simulink model "DOF4_model_v2"  (R2023a)
settings: Solver=FixedStepAuto  StartTime=0.0  StopTime=10.0  FixedStep=5e-3  RelTol=1e-3
values from neighbouring files (symbols this model uses):
  z_r_type = 1    [DOF_4_parameters.m]
undefined symbols (not defined in the file or in its folder): chassis, constants, suspension
libraries: simulink x1
settings Model: Creator=Cassio de Freitas  LastModifiedBy=Cassio de Freitas
settings DataIOCC: ReturnWorkspaceOutputsName=simout

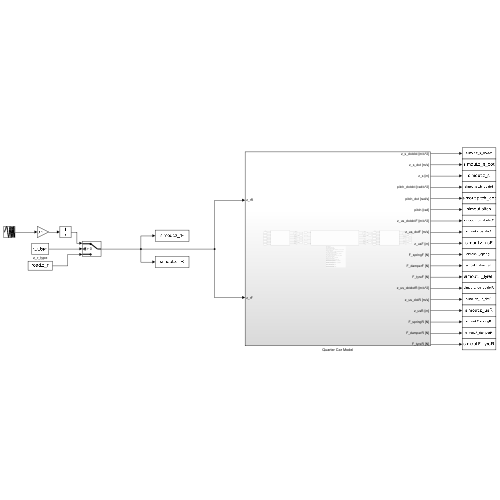
[thumbnail: Simulink's stored preview of the top-level diagram]
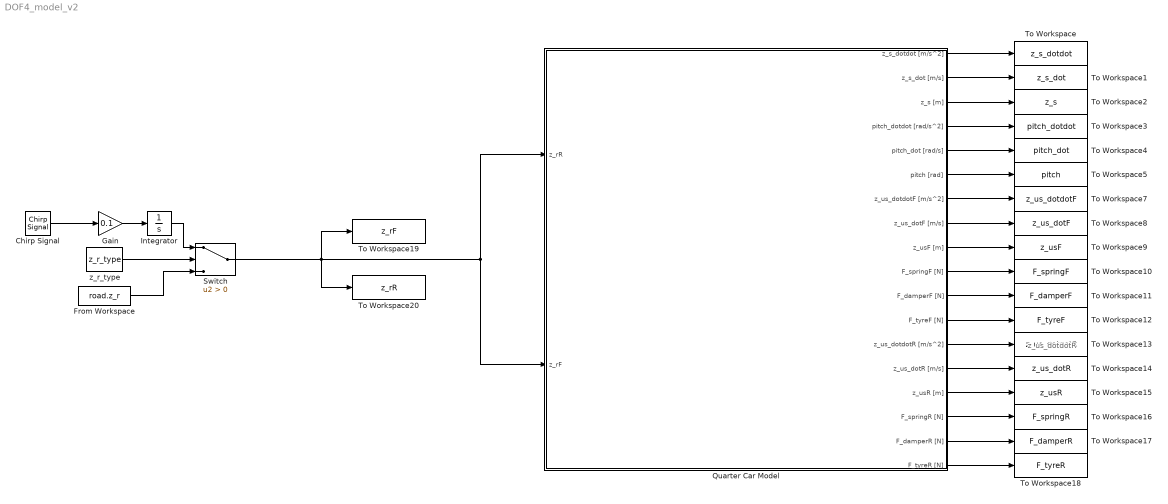
== system DOF4_model_v2 ==
  note: z_us_dotdotR
  Chirp Signal : simulink/Sources/Chirp Signal  f1=0.1  T=100  f2=50
  From Workspace : FromWorkspace  VariableName=road.z_r
  Gain : Gain  Gain=0.1
  Integrator : Integrator
  Quarter Car Model : Subsystem
  Switch : Switch  Criteria=u2 > Threshold  SaturateOnIntegerOverflow=off  InputSameDT=off
  To Workspace : ToWorkspace  VariableName=z_s_dotdot  SaveFormat=Timeseries  SampleTime=-1
  To Workspace1 : ToWorkspace  VariableName=z_s_dot  SaveFormat=Timeseries  SampleTime=-1
  To Workspace10 : ToWorkspace  VariableName=F_springF  SaveFormat=Timeseries  SampleTime=-1
  To Workspace11 : ToWorkspace  VariableName=F_damperF  SaveFormat=Timeseries  SampleTime=-1
  To Workspace12 : ToWorkspace  VariableName=F_tyreF  SaveFormat=Timeseries  SampleTime=-1
  To Workspace13 : ToWorkspace  VariableName=z_us_dotdotR  SaveFormat=Timeseries  SampleTime=-1
  To Workspace14 : ToWorkspace  VariableName=z_us_dotR  SaveFormat=Timeseries  SampleTime=-1
  To Workspace15 : ToWorkspace  VariableName=z_usR  SaveFormat=Timeseries  SampleTime=-1
  To Workspace16 : ToWorkspace  VariableName=F_springR  SaveFormat=Timeseries  SampleTime=-1
  To Workspace17 : ToWorkspace  VariableName=F_damperR  SaveFormat=Timeseries  SampleTime=-1
  To Workspace18 : ToWorkspace  VariableName=F_tyreR  SaveFormat=Timeseries  SampleTime=-1
  To Workspace19 : ToWorkspace  VariableName=z_rF  SaveFormat=Timeseries  SampleTime=-1
  To Workspace2 : ToWorkspace  VariableName=z_s  SaveFormat=Timeseries  SampleTime=-1
  To Workspace20 : ToWorkspace  VariableName=z_rR  SaveFormat=Timeseries  SampleTime=-1
  To Workspace3 : ToWorkspace  VariableName=pitch_dotdot  SaveFormat=Timeseries  SampleTime=-1
  To Workspace4 : ToWorkspace  VariableName=pitch_dot  SaveFormat=Timeseries  SampleTime=-1
  To Workspace5 : ToWorkspace  VariableName=pitch  SaveFormat=Timeseries  SampleTime=-1
  To Workspace7 : ToWorkspace  VariableName=z_us_dotdotF  SaveFormat=Timeseries  SampleTime=-1
  To Workspace8 : ToWorkspace  VariableName=z_us_dotF  SaveFormat=Timeseries  SampleTime=-1
  To Workspace9 : ToWorkspace  VariableName=z_usF  SaveFormat=Timeseries  SampleTime=-1
  z_r_type : Constant  Value=z_r_type
  wires:
  Integrator/1 -> Switch/1
  Gain/1 -> Integrator/1
  From Workspace/1 -> Switch/3
  z_r_type/1 -> Switch/2
  Chirp Signal/1 -> Gain/1
  Quarter Car Model/1(z_s_dotdot [m/s^2]) -> To Workspace/1
  Quarter Car Model/2(z_s_dot [m/s]) -> To Workspace1/1
  Quarter Car Model/3(z_s [m]) -> To Workspace2/1
  Quarter Car Model/4(pitch_dotdot [rad/s^2]) -> To Workspace3/1
  Quarter Car Model/5(pitch_dot [rad/s]) -> To Workspace4/1
  Quarter Car Model/6(pitch [rad]) -> To Workspace5/1
  Quarter Car Model/7(z_us_dotdotF [m/s^2]) -> To Workspace7/1
  Quarter Car Model/8(z_us_dotF [m/s]) -> To Workspace8/1
  Quarter Car Model/9(z_usF [m]) -> To Workspace9/1
  Quarter Car Model/10(F_springF [N]) -> To Workspace10/1
  Quarter Car Model/11(F_damperF [N]) -> To Workspace11/1
  Quarter Car Model/12(F_tyreF [N]) -> To Workspace12/1
  Quarter Car Model/13(z_us_dotdotR [m/s^2]) -> To Workspace13/1
  Quarter Car Model/14(z_us_dotR [m/s]) -> To Workspace14/1
  Quarter Car Model/15(z_usR [m]) -> To Workspace15/1
  Quarter Car Model/16(F_springR [N]) -> To Workspace16/1
  Quarter Car Model/17(F_damperR [N]) -> To Workspace17/1
  Quarter Car Model/18(F_tyreR [N]) -> To Workspace18/1
  Switch/1 -> To Workspace20/1, To Workspace19/1, Quarter Car Model/1(z_rR), Quarter Car Model/2(z_rF)

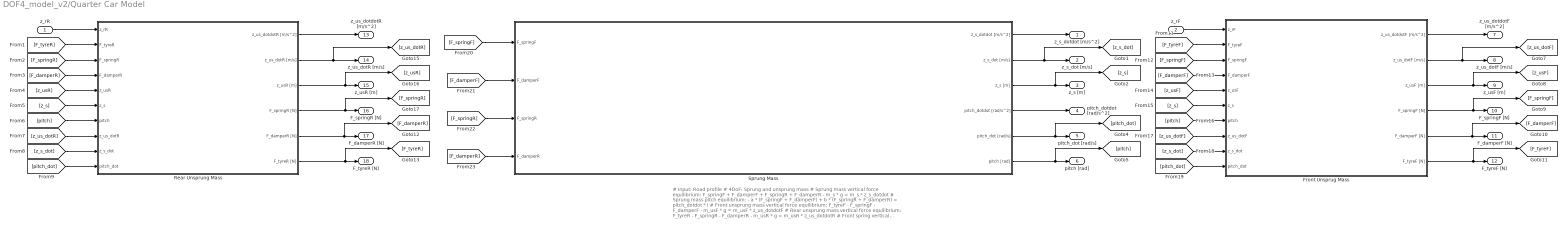
== system DOF4_model_v2/Quarter Car Model ==
  note: # Input: Road profile
      |
      | # 4DoF: Sprung and unsprung mass
      |
      | # Sprung mass vertical force equilibrium:
      | F_springF + F_damperF + F_springR + F_damperR - m_s * g = m_s * z_s_dotdot
      |
      | # Sprung mass pitch equilibrium:
      | - a * (F_springF + F_damperF) + b * (F_springR + F_damperR) = pitch_dotdot * I
      |
      | # Front unsprung mass vertical force equilibrium:
      | F_tyreF - F_springF - F_damperF - m_usF * g = m_usF * z_us_dotdotF
      |
      | # Rear unsprung mass vertical force equilibrium:
      | F_tyreR - F_springR - F_damperR - m_usR * g = m_usR * z_us_dotdotR
      |
      | # Front spring vertical force equilibrium
      | F_springF = (z_usF - (z_s - pitch * a)) * k_springF + F0F
      |
      | # Rear spring vertical force equilibrium
      | F_springR = (z_usR - (z_s + pitch * b)) * k_springR + F0R
      |
      | # Front damper vertical force equilibrium
      | F_damperF = (z_us_dotF - (z_s_dot - pitch_dot * a)) * c_damperF
      |
      | # Rear damper vertical force equilibrium
      | F_damperR = (z_us_dotR - (z_s_dot + pitch_dot * a)) * c_damperR
      |
      | # Front tyre vertical force equilibrium
      | F_tyreF = (z_rF - z_usF +z0_tyreF) * k_tyreF
      |
      | # Rear tyre vertical force equilibrium
      | F_tyreR = (z_rR - z_usR +z0_tyreR) * k_tyreR
  z_rR : Inport
  z_rF : Inport  Port=2
  Front Unsprug Mass : Subsystem
  Rear Unsprung Mass : Subsystem
  Sprung Mass : Subsystem
  z_s_dotdot [m/s^2] : Outport
  z_s_dot [m/s] : Outport  Port=2
  z_s [m] : Outport  Port=3
  pitch_dotdot [rad/s^2] : Outport  Port=4
  pitch_dot [rad/s] : Outport  Port=5
  pitch [rad] : Outport  Port=6
  z_us_dotdotF [m/s^2] : Outport  Port=7
  z_us_dotF [m/s] : Outport  Port=8
  z_usF [m] : Outport  Port=9
  F_springF [N] : Outport  Port=10
  F_damperF [N] : Outport  Port=11
  F_tyreF [N] : Outport  Port=12
  z_us_dotdotR [m/s^2] : Outport  Port=13
  z_us_dotR [m/s] : Outport  Port=14
  z_usR [m] : Outport  Port=15
  F_springR [N] : Outport  Port=16
  F_damperR [N] : Outport  Port=17
  F_tyreR [N] : Outport  Port=18
  wires:
  Sprung Mass/1(z_s_dotdot [m/s^2]) -> z_s_dotdot [m/s^2]/1
  Sprung Mass/2(z_s_dot [m/s]) -> z_s_dot [m/s]/1, [z_s_dot]
  Sprung Mass/3(z_s [m]) -> [z_s], z_s [m]/1
  Sprung Mass/4(pitch_dotdot [rad/s^2]) -> pitch_dotdot [rad/s^2]/1
  Sprung Mass/5(pitch_dot [rad/s]) -> [pitch_dot], pitch_dot [rad/s]/1
  Sprung Mass/6(pitch [rad]) -> [pitch], pitch [rad]/1
  Front Unsprug Mass/6(F_tyreF [N]) -> F_tyreF [N]/1, [F_tyreF]
  Front Unsprug Mass/5(F_damperF [N]) -> F_damperF [N]/1, [F_damperF]
  Front Unsprug Mass/4(F_springF [N]) -> F_springF [N]/1, [F_springF]
  Front Unsprug Mass/3(z_usF [m]) -> z_usF [m]/1, [z_usF]
  Front Unsprug Mass/2(z_us_dotF [m/s]) -> [z_us_dotF], z_us_dotF [m/s]/1
  Front Unsprug Mass/1(z_us_dotdotF [m/s^2]) -> z_us_dotdotF [m/s^2]/1
  Rear Unsprung Mass/3(z_usR [m]) -> z_usR [m]/1, [z_usR]
  Rear Unsprung Mass/4(F_springR [N]) -> F_springR [N]/1, [F_springR]
  Rear Unsprung Mass/5(F_damperR [N]) -> F_damperR [N]/1, [F_damperR]
  Rear Unsprung Mass/2(z_us_dotR [m/s]) -> [z_us_dotR], z_us_dotR [m/s]/1
  Rear Unsprung Mass/6(F_tyreR [N]) -> F_tyreR [N]/1, [F_tyreR]
  Rear Unsprung Mass/1(z_us_dotdotR [m/s^2]) -> z_us_dotdotR [m/s^2]/1
  z_rR/1 -> Rear Unsprung Mass/1(z_rR)
  [pitch_dot] -> Rear Unsprung Mass/10(pitch_dot)
  [z_s_dot] -> Rear Unsprung Mass/9(z_s_dot)
  [z_us_dotR] -> Rear Unsprung Mass/8(z_us_dotR)
  [pitch] -> Rear Unsprung Mass/7(pitch)
  [z_s] -> Rear Unsprung Mass/6(z_s)
  [z_usR] -> Rear Unsprung Mass/5(z_usR)
  [F_damperR] -> Rear Unsprung Mass/4(F_damperR)
  [F_springR] -> Rear Unsprung Mass/3(F_springR)
  [F_tyreR] -> Rear Unsprung Mass/2(F_tyreR)
  [F_damperF] -> Front Unsprug Mass/4(F_damperF)
  [z_us_dotF] -> Front Unsprug Mass/8(z_us_dotF)
  [z_s_dot] -> Front Unsprug Mass/9(z_s_dot)
  z_rF/1 -> Front Unsprug Mass/1(z_rF)
  [F_tyreF] -> Front Unsprug Mass/2(F_tyreF)
  [pitch] -> Front Unsprug Mass/7(pitch)
  [z_s] -> Front Unsprug Mass/6(z_s)
  [F_springF] -> Front Unsprug Mass/3(F_springF)
  [z_usF] -> Front Unsprug Mass/5(z_usF)
  [pitch_dot] -> Front Unsprug Mass/10(pitch_dot)
  [F_springF] -> Sprung Mass/1(F_springF)
  [F_damperF] -> Sprung Mass/2(F_damperF)
  [F_springR] -> Sprung Mass/3(F_springR)
  [F_damperR] -> Sprung Mass/4(F_damperR)

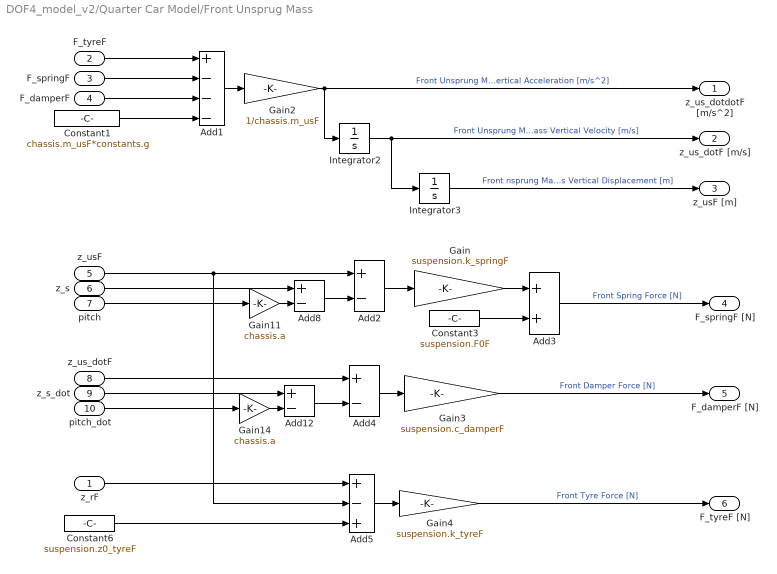
== system DOF4_model_v2/Quarter Car Model/Front Unsprug Mass ==
  z_rF : Inport
  F_tyreF : Inport  Port=2
  F_springF : Inport  Port=3
  F_damperF : Inport  Port=4
  z_usF : Inport  Port=5
  z_s : Inport  Port=6
  pitch : Inport  Port=7
  z_us_dotF : Inport  Port=8
  z_s_dot : Inport  Port=9
  pitch_dot : Inport  Port=10
  Add1 : Sum  Inputs=+---
  Add{2,4,8,12} (4 alike) : Sum  Inputs=+-
  Add3 : Sum
  Add5 : Sum  Inputs=+-+
  Constant1 : Constant  Value=chassis.m_usF*constants.g
  Constant3 : Constant  Value=suspension.F0F
  Constant6 : Constant  Value=suspension.z0_tyreF
  Gain : Gain  Gain=suspension.k_springF
  Gain11 : Gain  Gain=chassis.a
  Gain14 : Gain  Gain=chassis.a
  Gain2 : Gain  Gain=1/chassis.m_usF
  Gain3 : Gain  Gain=suspension.c_damperF
  Gain4 : Gain  Gain=suspension.k_tyreF
  Integrator2 : Integrator
  Integrator3 : Integrator
  z_us_dotdotF [m/s^2] : Outport
  z_us_dotF [m/s] : Outport  Port=2
  z_usF [m] : Outport  Port=3
  F_springF [N] : Outport  Port=4
  F_damperF [N] : Outport  Port=5
  F_tyreF [N] : Outport  Port=6
  wires:
  Integrator3/1 -> z_usF [m]/1  "Front nsprung Mass Vertical Displacement [m]"
  Add1/1 -> Gain2/1
  Integrator2/1 -> z_us_dotF [m/s]/1, Integrator3/1  "Front Unsprung Mass Vertical Velocity [m/s]"
  Gain2/1 -> Integrator2/1, z_us_dotdotF [m/s^2]/1  "Front Unsprung Mass Vertical Acceleration [m/s^2]"
  Gain11/1 -> Add8/2
  z_s/1 -> Add8/1
  Add8/1 -> Add2/2
  Add3/1 -> F_springF [N]/1  "Front Spring Force [N]"
  Gain/1 -> Add3/1
  Add4/1 -> Gain3/1
  Constant3/1 -> Add3/2
  z_usF/1 -> Add5/2, Add2/1
  Gain3/1 -> F_damperF [N]/1  "Front Damper Force [N]"
  Gain14/1 -> Add12/2
  pitch/1 -> Gain11/1
  Add2/1 -> Gain/1
  Add12/1 -> Add4/2
  Add5/1 -> Gain4/1
  z_rF/1 -> Add5/1
  Constant6/1 -> Add5/3
  Gain4/1 -> F_tyreF [N]/1  "Front Tyre Force [N]"
  F_damperF/1 -> Add1/3
  F_tyreF/1 -> Add1/1
  F_springF/1 -> Add1/2
  Constant1/1 -> Add1/4
  z_us_dotF/1 -> Add4/1
  z_s_dot/1 -> Add12/1
  pitch_dot/1 -> Gain14/1

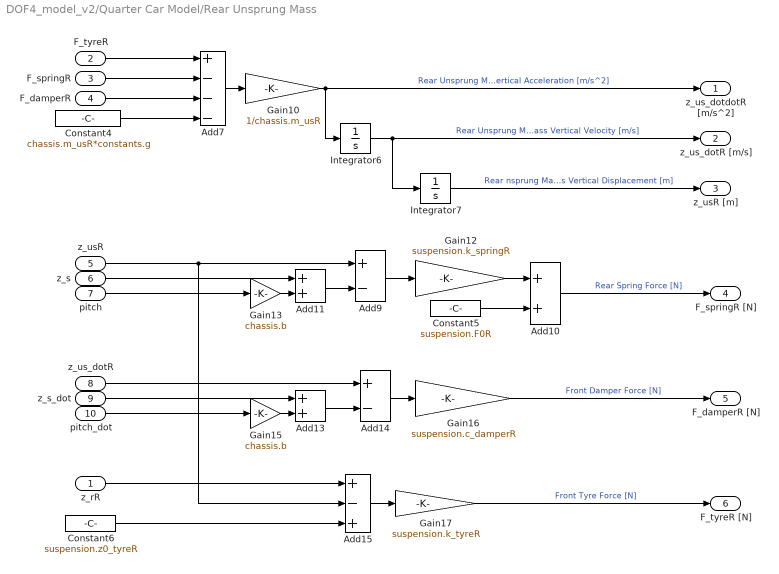
== system DOF4_model_v2/Quarter Car Model/Rear Unsprung Mass ==
  z_rR : Inport
  F_tyreR : Inport  Port=2
  F_springR : Inport  Port=3
  F_damperR : Inport  Port=4
  z_usR : Inport  Port=5
  z_s : Inport  Port=6
  pitch : Inport  Port=7
  z_us_dotR : Inport  Port=8
  z_s_dot : Inport  Port=9
  pitch_dot : Inport  Port=10
  Add10 : Sum
  Add11 : Sum
  Add13 : Sum
  Add14 : Sum  Inputs=+-
  Add15 : Sum  Inputs=+-+
  Add7 : Sum  Inputs=+---
  Add9 : Sum  Inputs=+-
  Constant4 : Constant  Value=chassis.m_usR*constants.g
  Constant5 : Constant  Value=suspension.F0R
  Constant6 : Constant  Value=suspension.z0_tyreR
  Gain10 : Gain  Gain=1/chassis.m_usR
  Gain12 : Gain  Gain=suspension.k_springR
  Gain13 : Gain  Gain=chassis.b
  Gain15 : Gain  Gain=chassis.b
  Gain16 : Gain  Gain=suspension.c_damperR
  Gain17 : Gain  Gain=suspension.k_tyreR
  Integrator6 : Integrator
  Integrator7 : Integrator
  z_us_dotdotR [m/s^2] : Outport
  z_us_dotR [m/s] : Outport  Port=2
  z_usR [m] : Outport  Port=3
  F_springR [N] : Outport  Port=4
  F_damperR [N] : Outport  Port=5
  F_tyreR [N] : Outport  Port=6
  wires:
  Integrator7/1 -> z_usR [m]/1  "Rear nsprung Mass Vertical Displacement [m]"
  Add7/1 -> Gain10/1
  Gain10/1 -> Integrator6/1, z_us_dotdotR [m/s^2]/1  "Rear Unsprung Mass Vertical Acceleration [m/s^2]"
  Integrator6/1 -> z_us_dotR [m/s]/1, Integrator7/1  "Rear Unsprung Mass Vertical Velocity [m/s]"
  Add11/1 -> Add9/2
  Add9/1 -> Gain12/1
  Gain16/1 -> F_damperR [N]/1  "Front Damper Force [N]"
  Add13/1 -> Add14/2
  Gain13/1 -> Add11/2
  Gain12/1 -> Add10/1
  Add14/1 -> Gain16/1
  Add10/1 -> F_springR [N]/1  "Rear Spring Force [N]"
  Gain15/1 -> Add13/2
  Constant5/1 -> Add10/2
  Gain17/1 -> F_tyreR [N]/1  "Front Tyre Force [N]"
  Add15/1 -> Gain17/1
  F_tyreR/1 -> Add7/1
  F_springR/1 -> Add7/2
  F_damperR/1 -> Add7/3
  Constant4/1 -> Add7/4
  z_usR/1 -> Add15/2, Add9/1
  z_s/1 -> Add11/1
  pitch/1 -> Gain13/1
  z_us_dotR/1 -> Add14/1
  z_s_dot/1 -> Add13/1
  pitch_dot/1 -> Gain15/1
  z_rR/1 -> Add15/1
  Constant6/1 -> Add15/3

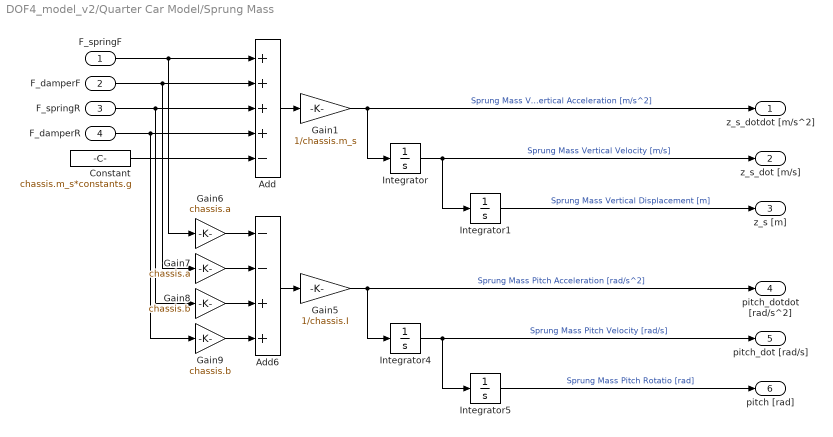
== system DOF4_model_v2/Quarter Car Model/Sprung Mass ==
  F_springF : Inport
  F_damperF : Inport  Port=2
  F_springR : Inport  Port=3
  F_damperR : Inport  Port=4
  Add : Sum  Inputs=++++-
  Add6 : Sum  Inputs=--++
  Constant : Constant  Value=chassis.m_s*constants.g
  Gain1 : Gain  Gain=1/chassis.m_s
  Gain5 : Gain  Gain=1/chassis.I
  Gain6 : Gain  Gain=chassis.a
  Gain7 : Gain  Gain=chassis.a
  Gain8 : Gain  Gain=chassis.b
  Gain9 : Gain  Gain=chassis.b
  Integrator{,1,4..5} (4 alike) : Integrator
  z_s_dotdot [m/s^2] : Outport
  z_s_dot [m/s] : Outport  Port=2
  z_s [m] : Outport  Port=3
  pitch_dotdot [rad/s^2] : Outport  Port=4
  pitch_dot [rad/s] : Outport  Port=5
  pitch [rad] : Outport  Port=6
  wires:
  Integrator4/1 -> pitch_dot [rad/s]/1, Integrator5/1  "Sprung Mass Pitch Velocity [rad/s]"
  Gain5/1 -> pitch_dotdot [rad/s^2]/1, Integrator4/1  "Sprung Mass Pitch Acceleration [rad/s^2]"
  Gain9/1 -> Add6/4
  Gain1/1 -> Integrator/1, z_s_dotdot [m/s^2]/1  "Sprung Mass Vertical Acceleration [m/s^2]"
  Integrator1/1 -> z_s [m]/1  "Sprung Mass Vertical Displacement [m]"
  Add/1 -> Gain1/1
  Gain8/1 -> Add6/3
  Add6/1 -> Gain5/1
  Gain7/1 -> Add6/2
  Gain6/1 -> Add6/1
  Integrator5/1 -> pitch [rad]/1  "Sprung Mass Pitch Rotatio [rad]"
  Integrator/1 -> Integrator1/1, z_s_dot [m/s]/1  "Sprung Mass Vertical Velocity [m/s]"
  F_springF/1 -> Gain6/1, Add/1
  F_damperF/1 -> Gain7/1, Add/2
  F_springR/1 -> Gain8/1, Add/3
  F_damperR/1 -> Gain9/1, Add/4
  Constant/1 -> Add/5
